simulink model "AW_test"  (Simulink 7.1)
settings: Solver=ode5  StartTime=0.0  StopTime=0.5  FixedStep=1e-4  MaxStep=5e-5  MinStep=1e-14  RelTol=1e-12  AbsTol=1e-12
values from neighbouring files (symbols this model uses):
  Ak = rlqg.A    [main_matlab.m]
  Ap = A    [main_matlab.m]    (also in plant.mat = [-15.9802071238 -2566.97948561 -96.8709621573 -60.7443875975)
  Bk = rlqg.B    [main_matlab.m]
  Bp = B    [main_matlab.m]
  Ck = rlqg.C    [main_matlab.m]
  Cp = C    [main_matlab.m]
  Dk = rlqg.D    [main_matlab.m]
  Dp = zeros(1,2)    [main_matlab.m]
  K = X1*Q^-1    [main_matlab.m]    (also in matlab.mat = [448.393946734 633.750487939 42.3087814135 63.1637386109 -29)
  L = X2*U^-1    [main_matlab.m]    (also in matlab.mat = [-0.0096486610976  0.00921474783824; 0.831783979809  -0.4838)
undefined symbols (not defined in the file or in its folder): Af, Bf, Cf, Hf
settings Model: Creator=p4wp4w  LastModifiedBy=Ablah
settings OptimizationCC: ExpressionDepthLimit=128  InitFltsAndDblsToZero=off
settings DebuggingCC: SolverPrmCheckMsg=none  FcnCallInpInsideContextMsg=Enable All  StateNameClashWarn=none  StrictBusMsg=ErrorLevel1
settings CodeAppCC: CustomSymbolStrType=$N$R$M_T
settings GRTTargetCC: TargetFunctionLibrary=C89/C90 (ANSI)  CPPClassGenCompliant=off

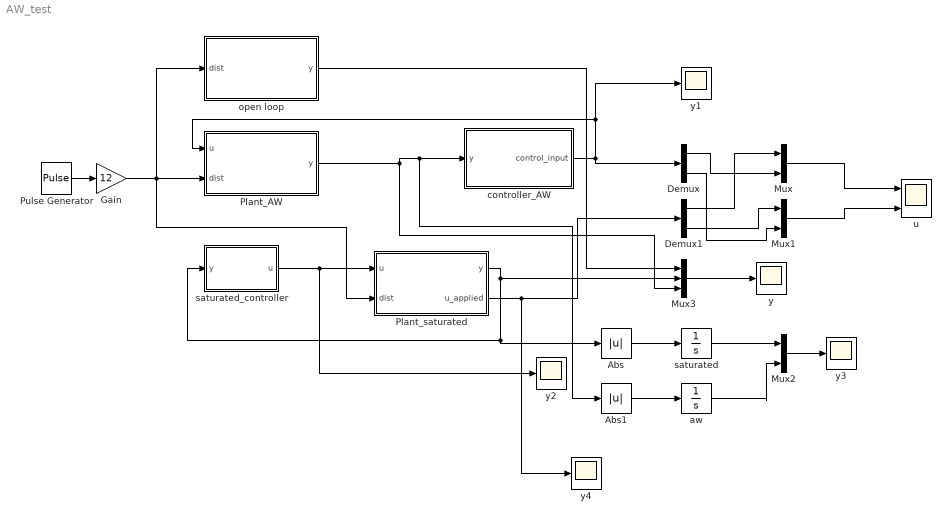
== system AW_test ==
  Abs : Abs
  Abs1 : Abs
  Demux : Demux  Outputs=2
  Demux1 : Demux  Outputs=2
  Gain : Gain  Gain=12
  Mux : Mux  Inputs=2
  Mux1 : Mux  Inputs=2
  Mux2 : Mux  Inputs=2
  Mux3 : Mux  Inputs=3
  Plant_AW : Subsystem
  Plant_saturated : Subsystem
  Pulse Generator : DiscretePulseGenerator  PulseType=Time based  Period=0.5  PulseWidth=10
  aw : Integrator
  controller_AW : Subsystem
  open loop : Subsystem
  saturated : Integrator
  "saturated_controller " : Subsystem
  u : Scope  NumInputPorts=2
      settings: YMin=-0.45~-0.2  YMax=0.2~0.125
  y{,1..4} (5 alike) : Scope
      y settings: YMin=-0.2  YMax=0.2
      y1 settings: SaveName=ScopeData4
      y2 settings: SaveName=ScopeData6
      y3 settings: SaveName=opt_out
      y4 settings: SaveName=ScopeData5
  wires:
  Plant_AW/1(y) -> Abs1/1, controller_AW/1(y), Mux3/3
  controller_AW/1("control_input ") -> y1/1, Plant_AW/1(u), Demux/1
  Pulse Generator/1 -> Gain/1
  Plant_saturated/1(y) -> Mux3/2, Abs/1, "saturated_controller "/1(y)
  Demux1/1 -> Mux/1
  Demux/1 -> Mux/2
  Demux1/2 -> Mux1/1
  Demux/2 -> Mux1/2
  Mux/1 -> u/1
  Mux1/1 -> u/2
  Plant_saturated/2(u_applied) -> y4/1, Demux1/1
  Gain/1 -> Plant_saturated/2(dist), open loop/1(dist), Plant_AW/2(dist)
  open loop/1(y) -> Mux3/1
  Mux3/1 -> y/1
  "saturated_controller "/1(u) -> y2/1, Plant_saturated/1(u)
  Mux2/1 -> y3/1
  saturated/1 -> Mux2/1
  aw/1 -> Mux2/2
  Abs/1 -> saturated/1
  Abs1/1 -> aw/1

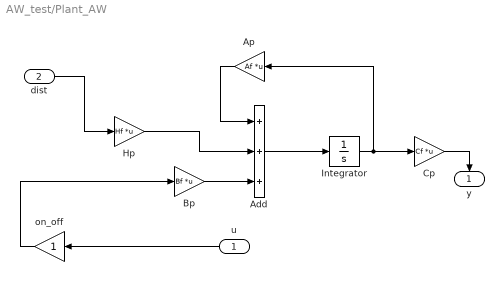
== system AW_test/Plant_AW ==
  u : Inport  Orientation=left
  dist : Inport  Port=2
  Add : Sum  Inputs=+++
  Ap : Gain  Orientation=left  Gain=Af  Multiplication=Matrix(K*u)
  Bp : Gain  Gain=Bf  Multiplication=Matrix(K*u)
  Cp : Gain  Gain=Cf  Multiplication=Matrix(K*u)
  Hp : Gain  Gain=Hf  Multiplication=Matrix(K*u)
  Integrator : Integrator
  on_off : Gain  Orientation=left
  y : Outport  Orientation=down
  wires:
  Add/1 -> Integrator/1
  Cp/1 -> y/1
  Hp/1 -> Add/2
  on_off/1 -> Bp/1
  Integrator/1 -> Cp/1, Ap/1
  u/1 -> on_off/1
  Ap/1 -> Add/1
  Bp/1 -> Add/3
  dist/1 -> Hp/1

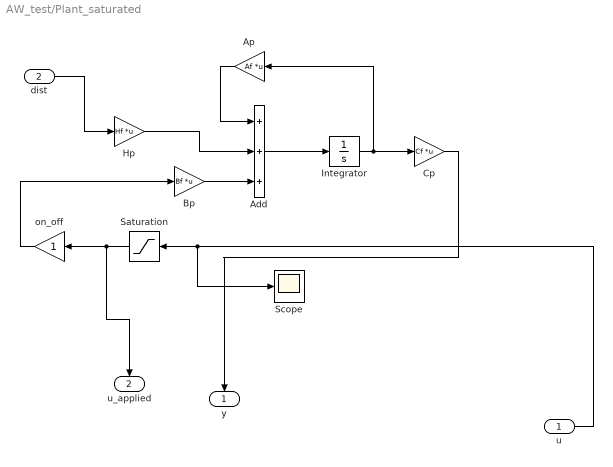
== system AW_test/Plant_saturated ==
  u : Inport
  dist : Inport  Port=2
  Add : Sum  Inputs=+++
  Ap : Gain  Orientation=left  Gain=Af  Multiplication=Matrix(K*u)
  Bp : Gain  Gain=Bf  Multiplication=Matrix(K*u)
  Cp : Gain  Gain=Cf  Multiplication=Matrix(K*u)
  Hp : Gain  Gain=Hf  Multiplication=Matrix(K*u)
  Integrator : Integrator
  Saturation : Saturate  Orientation=left  UpperLimit=2  LowerLimit=-2
  Scope : Scope
      settings: YMin=-10  YMax=10  SaveName=ScopeData2
  on_off : Gain  Orientation=left
  y : Outport  Orientation=down
  u_applied : Outport  Orientation=down  Port=2
  wires:
  dist/1 -> Hp/1
  Bp/1 -> Add/3
  u/1 -> Scope/1, Saturation/1
  Ap/1 -> Add/1
  Saturation/1 -> u_applied/1, on_off/1
  Integrator/1 -> Ap/1, Cp/1
  on_off/1 -> Bp/1
  Hp/1 -> Add/2
  Cp/1 -> y/1
  Add/1 -> Integrator/1

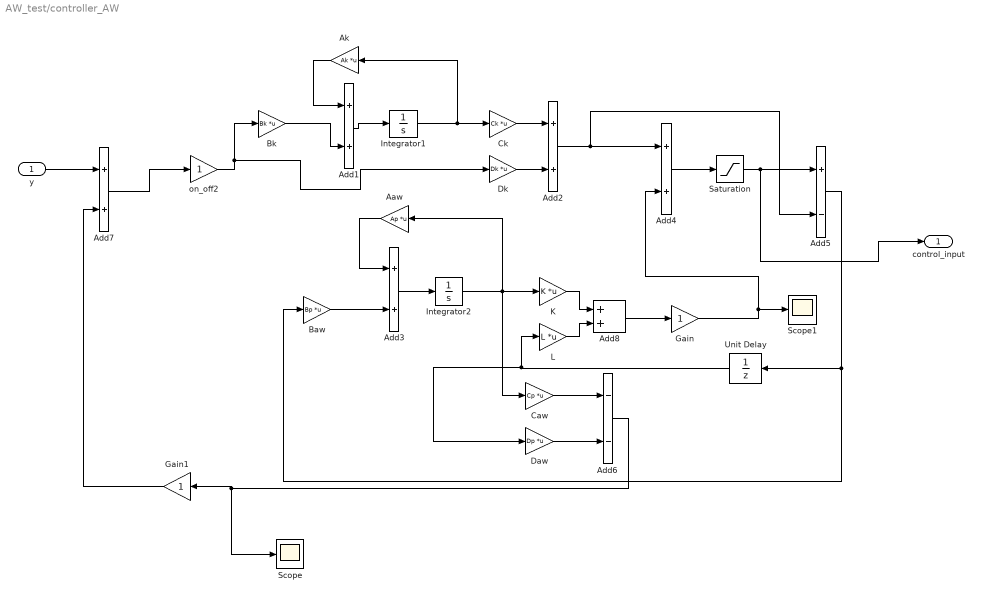
== system AW_test/controller_AW ==
  y : Inport
  Aaw : Gain  Orientation=left  Gain=Ap  Multiplication=Matrix(K*u)
  Add{1..4,7..8} (6 alike) : Sum
  Add5 : Sum  Inputs=+-
  Add6 : Sum  Inputs=--
  Ak : Gain  Orientation=left  Gain=Ak  Multiplication=Matrix(K*u)
  Baw : Gain  Gain=Bp  Multiplication=Matrix(K*u)
  Bk : Gain  Gain=Bk  Multiplication=Matrix(K*u)
  Caw : Gain  Gain=Cp  Multiplication=Matrix(K*u)
  Ck : Gain  Gain=Ck  Multiplication=Matrix(K*u)
  Daw : Gain  Gain=Dp  Multiplication=Matrix(K*u)
  Dk : Gain  Gain=Dk  Multiplication=Matrix(K*u)
  Gain : Gain
  Gain1 : Gain  Orientation=left
  Integrator1 : Integrator
  Integrator2 : Integrator
  K : Gain  Gain=K  Multiplication=Matrix(K*u)
  L : Gain  Gain=L  Multiplication=Matrix(K*u)
  Saturation : Saturate  UpperLimit=2  LowerLimit=-2
  Scope : Scope
      settings: SaveName=ScopeData3
  Scope1 : Scope
      settings: SaveName=ScopeData7
  Unit Delay : UnitDelay  Orientation=left  SampleTime=-1
  on_off2 : Gain
  "control_input " : Outport
  wires:
  Ck/1 -> Add2/1
  Add1/1 -> Integrator1/1
  Ak/1 -> Add1/1
  Bk/1 -> Add1/2
  Integrator1/1 -> Ck/1, Ak/1
  Dk/1 -> Add2/2
  on_off2/1 -> Dk/1, Bk/1
  Add3/1 -> Integrator2/1
  Aaw/1 -> Add3/1
  Baw/1 -> Add3/2
  Integrator2/1 -> Caw/1, K/1, Aaw/1
  Add2/1 -> Add5/2, Add4/1
  Add4/1 -> Saturation/1
  Saturation/1 -> "control_input "/1, Add5/1
  Caw/1 -> Add6/1
  Daw/1 -> Add6/2
  y/1 -> Add7/1
  Add7/1 -> on_off2/1
  K/1 -> Add8/1
  L/1 -> Add8/2
  Add8/1 -> Gain/1
  Add5/1 -> Baw/1, Unit Delay/1
  Unit Delay/1 -> L/1, Daw/1
  Add6/1 -> Gain1/1, Scope/1
  Gain/1 -> Scope1/1, Add4/2
  Gain1/1 -> Add7/2

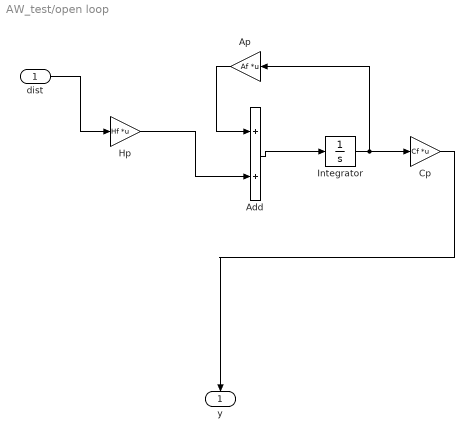
== system AW_test/open loop ==
  dist : Inport
  Add : Sum
  Ap : Gain  Orientation=left  Gain=Af  Multiplication=Matrix(K*u)
  Cp : Gain  Gain=Cf  Multiplication=Matrix(K*u)
  Hp : Gain  Gain=Hf  Multiplication=Matrix(K*u)
  Integrator : Integrator
  y : Outport  Orientation=down
  wires:
  dist/1 -> Hp/1
  Ap/1 -> Add/1
  Integrator/1 -> Ap/1, Cp/1
  Hp/1 -> Add/2
  Cp/1 -> y/1
  Add/1 -> Integrator/1

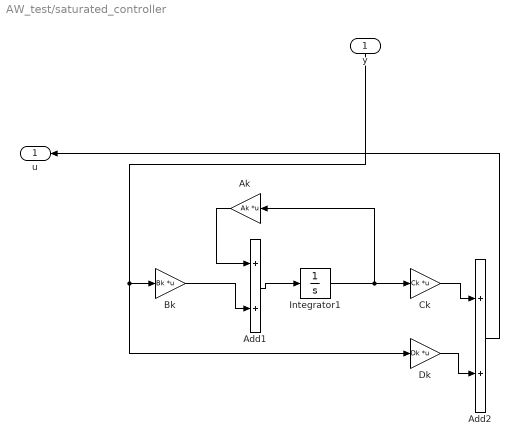
== system AW_test/saturated_controller  ==
  y : Inport  Orientation=down
  Add1 : Sum
  Add2 : Sum
  Ak : Gain  Orientation=left  Gain=Ak  Multiplication=Matrix(K*u)
  Bk : Gain  Gain=Bk  Multiplication=Matrix(K*u)
  Ck : Gain  Gain=Ck  Multiplication=Matrix(K*u)
  Dk : Gain  Gain=Dk  Multiplication=Matrix(K*u)
  Integrator1 : Integrator
  u : Outport  Orientation=left
  wires:
  Bk/1 -> Add1/2
  Add1/1 -> Integrator1/1
  Ck/1 -> Add2/1
  Dk/1 -> Add2/2
  Integrator1/1 -> Ck/1, Ak/1
  Add2/1 -> u/1
  Ak/1 -> Add1/1
  y/1 -> Bk/1, Dk/1
